simulink model "Lab_2_Simulink_Setup"  (R2023b)
settings: Solver=VariableStepAuto  StartTime=0.0  StopTime=inf  RelTol=1e-3
undefined symbols (not defined in the file or in its folder): CR, LF
libraries: instrumentseriallib x3
settings Model: Creator=blake  LastModifiedBy=blake

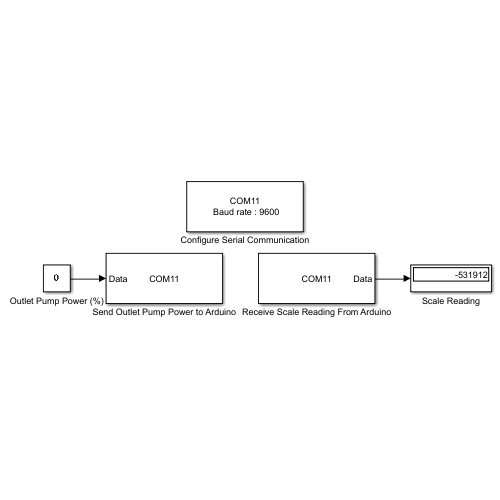
[thumbnail: Simulink's stored preview of the top-level diagram]
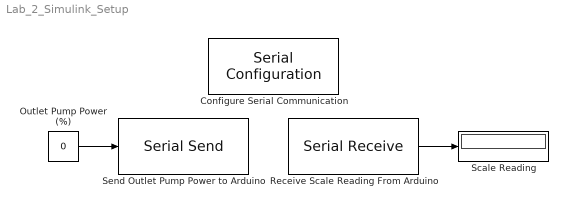
== system Lab_2_Simulink_Setup ==
  Configure Serial Communication : instrumentseriallib/Serial Configuration  Priority=-200000  PortSel=COM11  Port=COM11  ComPort=COM11  BaudRate=9600  DataBits=8  Parity=none  StopBits=1  ByteOrder=little-endian  FlowControl=none  Timeout=1  SimulateUsing=Interpreted execution  BlockInModel=on  aMode=1
  Outlet Pump Power (%) : Constant  Value=0  OutDataTypeStr=single  SampleTime=0.05
  Receive Scale Reading From Arduino : instrumentseriallib/Serial Receive  Priority=1  PortSel=COM11  Port=COM11  ComPort=COM11  DataType=single  SaveDataType=uint8  ToggleHeader=off  Header=[]  DataSize=[1 1]  ToggleTerminator=on  Terminator=CR/LF ('\r\n')  CustomTerminator=[]  InputFormat=Column major  ToggleDataSize=on  EnableBlockingMode=on  ActionDataUnavailable=Output last received value  ActionWhenDataUnavailable=Output last received value  CustomValue=0  SampleTime=0.01  SimulateUsing=Interpreted execution  BlockInModel=on  aMode=1
  Scale Reading : Display
  Send Outlet Pump Power to Arduino : instrumentseriallib/Serial Send  Priority=1  PortSel=COM11  Port=COM11  ComPort=COM11  Header=[]  Terminator=CR/LF ('\r\n')  CustomTerminator=[]  EnableBlockingMode=on  SimulateUsing=Interpreted execution  BlockInModel=on  aMode=1
  wires:
  Receive Scale Reading From Arduino/1 -> Scale Reading/1
  Outlet Pump Power (%)/1 -> Send Outlet Pump Power to Arduino/1
